simulink model "distributive4"  (R2022b)
settings: Solver=ode8  StartTime=0.0  StopTime=0.25  FixedStep=0.0001  RelTol=1e-3
values from neighbouring files (symbols this model uses):
  A = [a11,0;0,a22]    [distributive3.m]    (also in neurobserver4.m = [1 1;1 2])
  alpha = 0.9e-6    (= 9e-07)    [distributive3.m]
  amp = 80e-6    (= 8e-05)    [distributive3.m]
  angvel = (2*pi)*30    (= 188.495559215)    [distributive3.m]
  B = [b11,0;0,b22]    [distributive3.m]    (also in neurobserver4.m = 1000)
  beta = 0.008    [distributive3.m]
  C = [1,0]    [distributive3.m]
  C_bar = [1,0]    [distributive3.m]    (also in neurobserver4.m = [1,0;0,1])
  d_p = 1.6e-6    (= 1.6e-06)    [distributive3.m]
  fase = 2*pi/10    (= 0.628318530718)    [distributive3.m]
  G = S\C_bar'    [distributive3.m]    (also in neurobserver4.m)
  gamma = 0.008    [distributive3.m]
  Gamma = [0,-B;0 0]    [distributive3.m]    (also in neurobserver4.m = [ 0 , -B ; 0 , 0 ])
  h = legend('Closed-loop response map $(y_d,y)$')    [distributive3.m]    (also in neurobserver4.m = legend('$(y_r,y)$ for $x=7.5$, $f=1Hz$','$(y_r,y)$ for $x=15)
  h_i = 2e-6    (= 2e-06)    [distributive3.m]
  k1 = 7    [distributive3.m]    (also in neurobserver4.m)
  k2 = 7    [distributive3.m]    (also in neurobserver4.m)
  kappa1 = 4e3    (= 4000)    [distributive3.m]    (also in neurobserver4.m = 120)
  L = 20000    [distributive3.m]
  S = [s11,s12;s21,s22]    [distributive3.m]    (also in neurobserver4.m = [1/theta,B/theta^2;B/theta^2,(2*B^2)/theta^3])
  V = learning.V    [neurobserver4.m]
  W = learning.W    [neurobserver4.m]
  x1 = e(2)    [distributive3.m]
  x2 = e(5)    [distributive3.m]
  y_i = -3e-6    (= -3e-06)    [distributive3.m]
undefined symbols (not defined in the file or in its folder): freq, Gamma_c, Y
(part 1 of 3)
settings Model: PacingRate=1000  Creator=mluser  LastModifiedBy=USER
settings OptimizationCC: EnhancedBackFolding=on  PassReuseOutputArgsThreshold=0  MaxStackSize=64  OptimizeBlockOrder=speed  DifferentSizesBufferReuse=on  OptimizationCustomize=off
settings DebuggingCC: SolverPrmCheckMsg=warning  ParameterTunabilityLossMsg=error  ModelReferenceExtraNoncontSigs=warning  UnderSpecifiedDimensionMsg=warning
settings HardwareCC: ProdBitPerPointer=32  ProdBitPerSizeT=32  ProdBitPerPtrDiffT=32  ProdLargestAtomicFloat=None  ProdIntDivRoundTo=Undefined  ProdEndianess=Unspecified  ProdWordSize=32  ProdHWDeviceType=Generic->Unspecified (assume 32-bit Generic)
settings ModelReferenceCC: EnableRefExpFcnMdlSchedulingChecks=on
settings SFSimCC: MATLABDynamicMemAlloc=off
settings RTWCC: Toolchain=Catkin
settings CodeAppCC: ForceParamTrailComments=on  OperatorAnnotations=on
settings GRTTargetCC: TargetLangStandard=C89/C90 (ANSI)

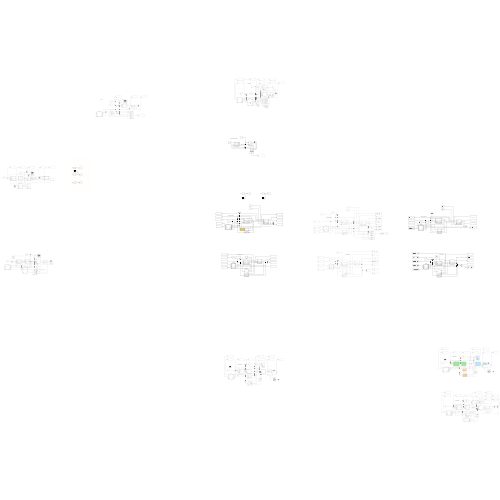
[thumbnail: Simulink's stored preview of the top-level diagram]
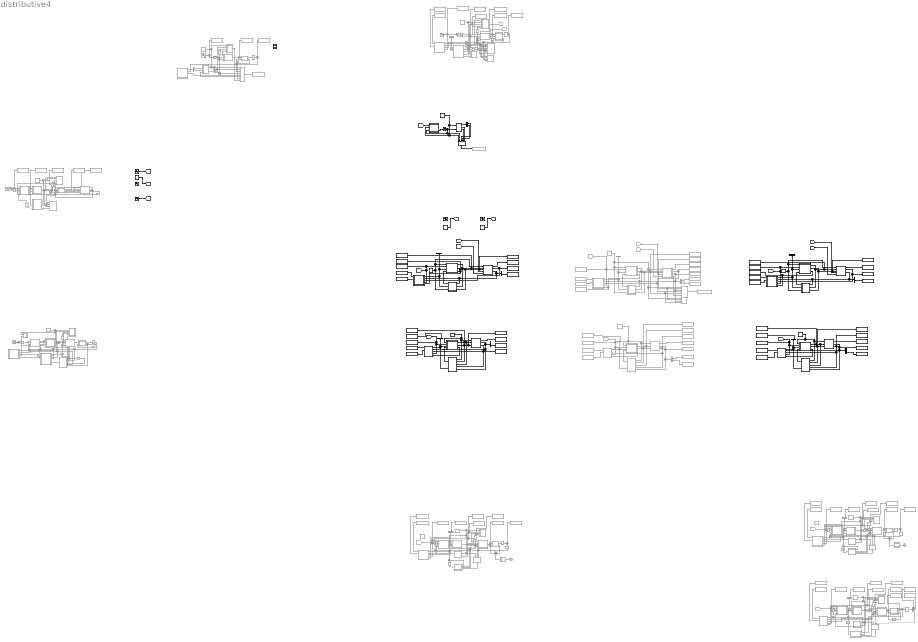
== system distributive4 ==
  note: model
  note: high gain observer
  note: neuroobserver
  note: neuroobserver
  note: inverse model controller
  note: neuroobserver
  note: neuroobserver
  note: no controller
  note: neuroobserver
  note: high gain observer
  note: neuroobserver
  note: high gain observer
  Clock : Clock  Commented=on
  Clock1 : Clock  Commented=on
  Delay3 : Delay  Commented=on  DelayLength=1  InitialCondition=0
  Delay4 : Delay  Commented=on  DelayLength=1  InitialCondition=0
  Demux{1,4,7,10..12,15,21,28} (9 alike) : Demux  Outputs=2
  Demux{2..3,5..6,8..9,23..24,27} (9 alike) : Demux  Commented=on  Outputs=2
  Derivative{2..3,7,12,29..31,35,37} (9 alike) : Derivative  Commented=on
  From1 : From  Commented=on  GotoTag=f10
  From19 : From  Commented=on  GotoTag=A1
  From2 : From  Commented=on  GotoTag=f10
  From21 : From  Commented=on  GotoTag=n
  From22 : From  Commented=on  GotoTag=ny
  From3 : From  Commented=on  GotoTag=ny
  From5 : From  Commented=on  GotoTag=n
  From8 : From  Commented=on  GotoTag=A1
  From9 : From  Commented=on  GotoTag=A1
  IC10 : InitialCondition  Commented=on  Value=0
  IC11 : InitialCondition  Commented=on  Value=h
  IC12 : InitialCondition  Commented=on  Value=Y
  IC13 : InitialCondition  Commented=on  Value=d_p
  IC{6,18..19,33..34} (5 alike) : InitialCondition  Commented=on  Value=h_i
  IC4 : InitialCondition  Commented=on  Value=h
  IC7 : InitialCondition  Commented=on  Value=y_i
  Integrator{2,22,24,35,39} (5 alike) : Integrator  Commented=on  InitialCondition=[0;0]
  Integrator{3,7..9,23,25,36,40} (8 alike) : Integrator  Commented=on
  L1 : Constant  Commented=on  Value=15000
  L5 : Constant  Value=x1
  Mux{1,4,7,23} (4 alike) : Mux  Commented=on  Inputs=8
      settings: DisplayOption=signals
  Mux17 : Mux  Commented=on  Inputs=3
      settings: DisplayOption=signals
  Mux19 : Mux  Commented=on  Inputs=3
      settings: DisplayOption=signals
  Mux2 : Mux  Inputs=6
  Mux22 : Mux  Commented=on  Inputs=3
      settings: DisplayOption=signals
  Mux3 : Mux  Commented=on
      settings: DisplayOption=signals
  Mux30 : Mux  Commented=on
      settings: DisplayOption=signals
  Mux6 : Mux  Commented=on  Inputs=2
  Saturation1 : Saturate  Commented=on  UpperLimit=2000  LowerLimit=-2000
  Saturation4 : Saturate  UpperLimit=20000  LowerLimit=-20000
  Signal Generator : SignalGenerator  WaveForm=sawtooth  Amplitude=amp  Frequency=angvel*10  Units=rad/sec
  Signal Generator1 : SignalGenerator  Amplitude=1*(1e-6)  Frequency=angvel*35  Units=rad/sec
  Signal Generator2 : SignalGenerator  Commented=on  Amplitude=amp  Frequency=angvel  Units=rad/sec
  Signal Generator3 : SignalGenerator  Commented=on  Amplitude=amp  Frequency=angvel  Units=rad/sec
  Signal Generator4 : SignalGenerator  WaveForm=random  Amplitude=1*(1e-6)  Frequency=angvel*20  Units=rad/sec
  Subsystem : Subsystem
  Subsystem1 : Subsystem  Commented=on
  Subsystem10 : Subsystem  Commented=on
  Subsystem11 : Subsystem  Commented=on
  Subsystem12 : Subsystem  Commented=on
      settings: PortSchema="{\"entries\":[{\"content\":{\"sides\":[{\"content\":{\"connectorIds\":[\"Out1\",\"Out2\",\"In1\"]},\"type\":\"ConnectorPlacement.EquallySpacedRectSide\",\"uuid\":\"42746eba-8bba-4a31-9528-796c8edd7bb7\"},{\"content\":{\"connectorIds\":[\"In2\",\"In3\",\"In4\"],\"side\":\"RIGHT\"},\"type\":\"ConnectorPlacement.EquallySpacedRectSide\",\"uuid\":\"7439d13e-5e36-47fa-9d41-de49a9f2c0eb\"},{\"content\":{\"connectorIds\":[],\"side\":\"TOP\"},\"type\":\"ConnectorPlacement.EquallySpacedRectSide\",\"uuid\":\"f708f9c0-884d-4497-944b-57601861f48d\"}]},\"type\":\"ConnectorPlacement.EquallySpacedConnector\",\"uuid\":\"a987a0bb-05be-4e20-b301-42abc30b9f40\"}],\"packageUris\":[\"http://schema.mathworks.com/mf0/Connector/R2020b\"],\"version\":\"1.0\"}"
  Subsystem13 : Subsystem
  Subsystem14 : Subsystem
  Subsystem15 : Subsystem
      settings: PortSchema="{\"entries\":[{\"content\":{\"sides\":[{\"content\":{\"connectorIds\":[\"Out1\",\"Out2\",\"In1\"]},\"type\":\"ConnectorPlacement.EquallySpacedRectSide\",\"uuid\":\"42746eba-8bba-4a31-9528-796c8edd7bb7\"},{\"content\":{\"connectorIds\":[\"In2\",\"In3\",\"In4\"],\"side\":\"RIGHT\"},\"type\":\"ConnectorPlacement.EquallySpacedRectSide\",\"uuid\":\"7439d13e-5e36-47fa-9d41-de49a9f2c0eb\"},{\"content\":{\"connectorIds\":[],\"side\":\"TOP\"},\"type\":\"ConnectorPlacement.EquallySpacedRectSide\",\"uuid\":\"f708f9c0-884d-4497-944b-57601861f48d\"}]},\"type\":\"ConnectorPlacement.EquallySpacedConnector\",\"uuid\":\"a987a0bb-05be-4e20-b301-42abc30b9f40\"}],\"packageUris\":[\"http://schema.mathworks.com/mf0/Connector/R2020b\"],\"version\":\"1.0\"}"
  Subsystem16 : Subsystem
  Subsystem17 : Subsystem
  Subsystem2 : Subsystem
  Subsystem3 : Subsystem
  Subsystem4 : Subsystem
  Subsystem5 : Subsystem
  Subsystem6 : Subsystem
  Subsystem7 : Subsystem
      settings: PortSchema="{\"entries\":[{\"content\":{\"sides\":[{\"content\":{\"connectorIds\":[\"Out1\",\"Out2\",\"In1\"]},\"type\":\"ConnectorPlacement.EquallySpacedRectSide\",\"uuid\":\"42746eba-8bba-4a31-9528-796c8edd7bb7\"},{\"content\":{\"connectorIds\":[\"In2\",\"In3\",\"In4\"],\"side\":\"RIGHT\"},\"type\":\"ConnectorPlacement.EquallySpacedRectSide\",\"uuid\":\"7439d13e-5e36-47fa-9d41-de49a9f2c0eb\"},{\"content\":{\"connectorIds\":[],\"side\":\"TOP\"},\"type\":\"ConnectorPlacement.EquallySpacedRectSide\",\"uuid\":\"f708f9c0-884d-4497-944b-57601861f48d\"}]},\"type\":\"ConnectorPlacement.EquallySpacedConnector\",\"uuid\":\"a987a0bb-05be-4e20-b301-42abc30b9f40\"}],\"packageUris\":[\"http://schema.mathworks.com/mf0/Connector/R2020b\"],\"version\":\"1.0\"}"
  Subsystem8 : Subsystem  Commented=on
  Subsystem9 : Subsystem  Commented=on
  Sum : Sum  Commented=on  Inputs=|++
  Sum1 : Sum  Commented=on  Inputs=|++
  To File1 : ToFile  Commented=on  Filename=train_f10_x1.mat  MatrixName=train
  To File3 : ToFile  Commented=on  Filename=train2_invmod_f1_x3.mat  MatrixName=train
  To File5 : ToFile  Commented=on  Filename=train_mod_20_10.mat  MatrixName=train
  To Workspace : ToWorkspace  Commented=on  VariableName=u_ref  SaveFormat=Timeseries  SampleTime=-1
  To Workspace1 : ToWorkspace  Commented=on  VariableName=y  SaveFormat=Timeseries  SampleTime=-1
  To Workspace10 : ToWorkspace  Commented=on  VariableName=upsilon  SaveFormat=Timeseries  SampleTime=-1
  To Workspace100 : ToWorkspace  Commented=on  VariableName=h_nn3  SaveFormat=Timeseries  SampleTime=-1
  To Workspace101 : ToWorkspace  Commented=on  VariableName=epsilon_y_nn2  SaveFormat=Timeseries  SampleTime=-1
  To Workspace102 : ToWorkspace  Commented=on  VariableName=epsilon_h_nn2  SaveFormat=Timeseries  SampleTime=-1
  To Workspace11 : ToWorkspace  Commented=on  VariableName=h_ref  SaveFormat=Timeseries  SampleTime=-1
  To Workspace12 : ToWorkspace  Commented=on  VariableName=y_ref  SaveFormat=Timeseries  SampleTime=-1
  To Workspace121 : ToWorkspace  VariableName=h_ref_nn3  SaveFormat=Timeseries  SampleTime=-1
  To Workspace122 : ToWorkspace  VariableName=y_ref_nn3  SaveFormat=Timeseries  SampleTime=-1
  To Workspace123 : ToWorkspace  VariableName=u_nn3  SaveFormat=Timeseries  SampleTime=-1
  To Workspace125 : ToWorkspace  VariableName=u_dot_nn3  SaveFormat=Timeseries  SampleTime=-1
  To Workspace126 : ToWorkspace  VariableName=h_nn3  SaveFormat=Timeseries  SampleTime=-1
  To Workspace127 : ToWorkspace  VariableName=epsilon_y_nn3  SaveFormat=Timeseries  SampleTime=-1
  To Workspace129 : ToWorkspace  VariableName=epsilon_h_nn3  SaveFormat=Timeseries  SampleTime=-1
  To Workspace13 : ToWorkspace  Commented=on  VariableName=h_nn  SaveFormat=Timeseries  SampleTime=-1
  To Workspace130 : ToWorkspace  VariableName=y_d_nn3  SaveFormat=Timeseries  SampleTime=-1
  To Workspace131 : ToWorkspace  Commented=on  VariableName=u_nn4  SaveFormat=Timeseries  SampleTime=-1
  To Workspace132 : ToWorkspace  Commented=on  VariableName=y_nn4  SaveFormat=Timeseries  SampleTime=-1
  To Workspace133 : ToWorkspace  Commented=on  VariableName=u_dot_nn4  SaveFormat=Timeseries  SampleTime=-1
  To Workspace135 : ToWorkspace  Commented=on  VariableName=h_nn4  SaveFormat=Timeseries  SampleTime=-1
  To Workspace136 : ToWorkspace  Commented=on  VariableName=epsilon_y_nn4  SaveFormat=Timeseries  SampleTime=-1
  To Workspace137 : ToWorkspace  Commented=on  VariableName=y_L_nn4  SaveFormat=Timeseries  SampleTime=-1
  To Workspace138 : ToWorkspace  Commented=on  VariableName=epsilon_h_nn4  SaveFormat=Timeseries  SampleTime=-1
  To Workspace139 : ToWorkspace  Commented=on  VariableName=y_d_nn4  SaveFormat=Timeseries  SampleTime=-1
  To Workspace14 : ToWorkspace  Commented=on  VariableName=epsilon_y_nn  SaveFormat=Timeseries  SampleTime=-1
  To Workspace140 : ToWorkspace  Commented=on  VariableName=upsilon_nn4  SaveFormat=Timeseries  SampleTime=-1
  To Workspace141 : ToWorkspace  Commented=on  VariableName=h_ref_nn4  SaveFormat=Timeseries  SampleTime=-1
  To Workspace142 : ToWorkspace  Commented=on  VariableName=y_ref_nn4  SaveFormat=Timeseries  SampleTime=-1
  To Workspace147 : ToWorkspace  Commented=on  VariableName=upsilon6  SaveFormat=Timeseries  SampleTime=-1
  To Workspace149 : ToWorkspace  Commented=on  VariableName=y_ref6  SaveFormat=Timeseries  SampleTime=-1
  To Workspace15 : ToWorkspace  Commented=on  VariableName=y_L_nn  SaveFormat=Timeseries  SampleTime=-1
  To Workspace150 : ToWorkspace  Commented=on  VariableName=u6  SaveFormat=Timeseries  SampleTime=-1
  To Workspace151 : ToWorkspace  Commented=on  VariableName=y6  SaveFormat=Timeseries  SampleTime=-1
  To Workspace152 : ToWorkspace  Commented=on  VariableName=u_dot6  SaveFormat=Timeseries  SampleTime=-1
  To Workspace153 : ToWorkspace  Commented=on  VariableName=h6  SaveFormat=Timeseries  SampleTime=-1
  To Workspace154 : ToWorkspace  Commented=on  VariableName=epsilon_y6  SaveFormat=Timeseries  SampleTime=-1
  To Workspace155 : ToWorkspace  Commented=on  VariableName=epsilon_h6  SaveFormat=Timeseries  SampleTime=-1
  To Workspace156 : ToWorkspace  VariableName=y_d_2  SaveFormat=Timeseries  SampleTime=-1
  To Workspace16 : ToWorkspace  Commented=on  VariableName=epsilon_h_nn  SaveFormat=Timeseries  SampleTime=-1
  To Workspace17 : ToWorkspace  Commented=on  VariableName=y_d_nn  SaveFormat=Timeseries  SampleTime=-1
  To Workspace18 : ToWorkspace  Commented=on  VariableName=y_L_nn1  SaveFormat=Timeseries  SampleTime=-1
  To Workspace19 : ToWorkspace  Commented=on  VariableName=y_d_nn1  SaveFormat=Timeseries  SampleTime=-1
  To Workspace2 : ToWorkspace  Commented=on  VariableName=upsilon  SaveFormat=Timeseries  SampleTime=-1
  To Workspace20 : ToWorkspace  Commented=on  VariableName=upsilon_nn  SaveFormat=Timeseries  SampleTime=-1
  To Workspace21 : ToWorkspace  Commented=on  VariableName=upsilon1  SaveFormat=Timeseries  SampleTime=-1
  To Workspace22 : ToWorkspace  Commented=on  VariableName=h_ref1  SaveFormat=Timeseries  SampleTime=-1
  To Workspace23 : ToWorkspace  Commented=on  VariableName=y_ref1  SaveFormat=Timeseries  SampleTime=-1
  To Workspace24 : ToWorkspace  Commented=on  VariableName=u1  SaveFormat=Timeseries  SampleTime=-1
  To Workspace25 : ToWorkspace  Commented=on  VariableName=y1  SaveFormat=Timeseries  SampleTime=-1
  To Workspace26 : ToWorkspace  Commented=on  VariableName=u_dot  SaveFormat=Timeseries  SampleTime=-1
  To Workspace27 : ToWorkspace  Commented=on  VariableName=h  SaveFormat=Timeseries  SampleTime=-1
  To Workspace28 : ToWorkspace  Commented=on  VariableName=epsilon_y  SaveFormat=Timeseries  SampleTime=-1
  To Workspace29 : ToWorkspace  Commented=on  VariableName=epsilon_h  SaveFormat=Timeseries  SampleTime=-1
  To Workspace3 : ToWorkspace  Commented=on  VariableName=h_ref_nn  SaveFormat=Timeseries  SampleTime=-1
  To Workspace30 : ToWorkspace  VariableName=h_nn4  SaveFormat=Timeseries  SampleTime=-1
  To Workspace31 : ToWorkspace  VariableName=epsilon_y_nn4  SaveFormat=Timeseries  SampleTime=-1
  To Workspace33 : ToWorkspace  VariableName=epsilon_h_nn4  SaveFormat=Timeseries  SampleTime=-1
  To Workspace34 : ToWorkspace  VariableName=y_d_nn4  SaveFormat=Timeseries  SampleTime=-1
  To Workspace36 : ToWorkspace  VariableName=y_d_3  SaveFormat=Timeseries  SampleTime=-1
  To Workspace37 : ToWorkspace  VariableName=upsilon_nn4  SaveFormat=Timeseries  SampleTime=-1
  To Workspace38 : ToWorkspace  VariableName=upsilon3  SaveFormat=Timeseries  SampleTime=-1
  To Workspace39 : ToWorkspace  VariableName=h_ref3  SaveFormat=Timeseries  SampleTime=-1
  To Workspace4 : ToWorkspace  Commented=on  VariableName=y_ref_nn  SaveFormat=Timeseries  SampleTime=-1
  To Workspace40 : ToWorkspace  VariableName=y_ref3  SaveFormat=Timeseries  SampleTime=-1
  To Workspace41 : ToWorkspace  VariableName=u3  SaveFormat=Timeseries  SampleTime=-1
  To Workspace43 : ToWorkspace  VariableName=u_dot3  SaveFormat=Timeseries  SampleTime=-1
  To Workspace44 : ToWorkspace  VariableName=h3  SaveFormat=Timeseries  SampleTime=-1
  To Workspace45 : ToWorkspace  VariableName=epsilon_y3  SaveFormat=Timeseries  SampleTime=-1
  To Workspace46 : ToWorkspace  VariableName=epsilon_h3  SaveFormat=Timeseries  SampleTime=-1
  To Workspace47 : ToWorkspace  VariableName=h_ref_nn4  SaveFormat=Timeseries  SampleTime=-1
  To Workspace48 : ToWorkspace  VariableName=upsilon_nn3  SaveFormat=Timeseries  SampleTime=-1
  To Workspace49 : ToWorkspace  VariableName=upsilon2  SaveFormat=Timeseries  SampleTime=-1
  To Workspace5 : ToWorkspace  Commented=on  VariableName=u_nn  SaveFormat=Timeseries  SampleTime=-1
  To Workspace50 : ToWorkspace  VariableName=h_ref2  SaveFormat=Timeseries  SampleTime=-1
  To Workspace51 : ToWorkspace  VariableName=y_ref2  SaveFormat=Timeseries  SampleTime=-1
  To Workspace52 : ToWorkspace  VariableName=u2  SaveFormat=Timeseries  SampleTime=-1
  To Workspace54 : ToWorkspace  VariableName=u_dot2  SaveFormat=Timeseries  SampleTime=-1
  To Workspace55 : ToWorkspace  VariableName=h2  SaveFormat=Timeseries  SampleTime=-1
  To Workspace56 : ToWorkspace  VariableName=epsilon_y2  SaveFormat=Timeseries  SampleTime=-1
  To Workspace57 : ToWorkspace  VariableName=epsilon_h2  SaveFormat=Timeseries  SampleTime=-1
  To Workspace58 : ToWorkspace  VariableName=y_ref_nn4  SaveFormat=Timeseries  SampleTime=-1
  To Workspace59 : ToWorkspace  VariableName=u_nn4  SaveFormat=Timeseries  SampleTime=-1
  To Workspace6 : ToWorkspace  Commented=on  VariableName=y_nn  SaveFormat=Timeseries  SampleTime=-1
  To Workspace60 : ToWorkspace  VariableName=y_nn4  SaveFormat=Timeseries  SampleTime=-1
  To Workspace61 : ToWorkspace  VariableName=u_dot_nn4  SaveFormat=Timeseries  SampleTime=-1
  To Workspace7 : ToWorkspace  Commented=on  VariableName=u_dot_nn  SaveFormat=Timeseries  SampleTime=-1
  To Workspace8 : ToWorkspace  Commented=on  VariableName=u  SaveFormat=Timeseries  SampleTime=-1
  To Workspace85 : ToWorkspace  Commented=on  VariableName=upsilon_nn2  SaveFormat=Timeseries  SampleTime=-1
  To Workspace86 : ToWorkspace  Commented=on  VariableName=h_ref_nn2  SaveFormat=Timeseries  SampleTime=-1
  To Workspace87 : ToWorkspace  Commented=on  VariableName=y_ref_nn2  SaveFormat=Timeseries  SampleTime=-1
  To Workspace88 : ToWorkspace  Commented=on  VariableName=u_nn2  SaveFormat=Timeseries  SampleTime=-1
  To Workspace89 : ToWorkspace  Commented=on  VariableName=y_nn2  SaveFormat=Timeseries  SampleTime=-1
  To Workspace9 : ToWorkspace  Commented=on  VariableName=y  SaveFormat=Timeseries  SampleTime=-1
  To Workspace90 : ToWorkspace  Commented=on  VariableName=u_dot_nn2  SaveFormat=Timeseries  SampleTime=-1
  To Workspace91 : ToWorkspace  Commented=on  VariableName=h_nn2  SaveFormat=Timeseries  SampleTime=-1
  To Workspace92 : ToWorkspace  Commented=on  VariableName=epsilon_y_nn3  SaveFormat=Timeseries  SampleTime=-1
  To Workspace93 : ToWorkspace  Commented=on  VariableName=epsilon_h_nn3  SaveFormat=Timeseries  SampleTime=-1
  To Workspace94 : ToWorkspace  Commented=on  VariableName=upsilon_nn3  SaveFormat=Timeseries  SampleTime=-1
  To Workspace95 : ToWorkspace  Commented=on  VariableName=h_ref_nn3  SaveFormat=Timeseries  SampleTime=-1
  To Workspace96 : ToWorkspace  Commented=on  VariableName=y_ref_nn3  SaveFormat=Timeseries  SampleTime=-1
  To Workspace97 : ToWorkspace  Commented=on  VariableName=u_nn3  SaveFormat=Timeseries  SampleTime=-1
  To Workspace98 : ToWorkspace  Commented=on  VariableName=y_nn3  SaveFormat=Timeseries  SampleTime=-1
  To Workspace99 : ToWorkspace  Commented=on  VariableName=u_dot_nn3  SaveFormat=Timeseries  SampleTime=-1
  dist_vars11 : Subsystem  Commented=on
      settings: PortSchema="{\"entries\":[{\"content\":{\"sides\":[{\"content\":{\"connectorIds\":[\"In1\",\"In2\",\"Out2\",\"Out3\"]},\"type\":\"ConnectorPlacement.EquallySpacedRectSide\",\"uuid\":\"c6804a03-85ed-4e19-a8b2-23b3b91cc999\"},{\"content\":{\"connectorIds\":[\"Out1\"],\"side\":\"RIGHT\"},\"type\":\"ConnectorPlacement.EquallySpacedRectSide\",\"uuid\":\"3893e005-dabd-44b9-aa2f-690b9b6a2b6d\"},{\"content\":{\"connectorIds\":[],\"side\":\"TOP\"},\"type\":\"ConnectorPlacement.EquallySpacedRectSide\",\"uuid\":\"9986ad97-c002-4a16-bb79-a95333cc5799\"}]},\"type\":\"ConnectorPlacement.EquallySpacedConnector\",\"uuid\":\"d796f436-4cc2-4114-998c-ef0d57f68d4d\"}],\"packageUris\":[\"http://schema.mathworks.com/mf0/Connector/R2020b\"],\"version\":\"1.0\"}"
  dist_vars22 : Subsystem  Commented=on
      settings: PortSchema="{\"entries\":[{\"content\":{\"sides\":[{\"content\":{\"connectorIds\":[\"Out1\",\"Out2\",\"Out3\"]},\"type\":\"ConnectorPlacement.EquallySpacedRectSide\",\"uuid\":\"c6804a03-85ed-4e19-a8b2-23b3b91cc999\"},{\"content\":{\"connectorIds\":[\"In1\",\"In2\"],\"side\":\"RIGHT\"},\"type\":\"ConnectorPlacement.EquallySpacedRectSide\",\"uuid\":\"3893e005-dabd-44b9-aa2f-690b9b6a2b6d\"},{\"content\":{\"connectorIds\":[],\"side\":\"TOP\"},\"type\":\"ConnectorPlacement.EquallySpacedRectSide\",\"uuid\":\"9986ad97-c002-4a16-bb79-a95333cc5799\"}]},\"type\":\"ConnectorPlacement.EquallySpacedConnector\",\"uuid\":\"d796f436-4cc2-4114-998c-ef0d57f68d4d\"}],\"packageUris\":[\"http://schema.mathworks.com/mf0/Connector/R2020b\"],\"version\":\"1.0\"}"
  dist_vars23 : Subsystem  Commented=on
      settings: PortSchema="{\"entries\":[{\"content\":{\"sides\":[{\"content\":{\"connectorIds\":[\"Out1\",\"Out2\",\"Out3\"]},\"type\":\"ConnectorPlacement.EquallySpacedRectSide\",\"uuid\":\"c6804a03-85ed-4e19-a8b2-23b3b91cc999\"},{\"content\":{\"connectorIds\":[\"In1\",\"In2\"],\"side\":\"RIGHT\"},\"type\":\"ConnectorPlacement.EquallySpacedRectSide\",\"uuid\":\"3893e005-dabd-44b9-aa2f-690b9b6a2b6d\"},{\"content\":{\"connectorIds\":[],\"side\":\"TOP\"},\"type\":\"ConnectorPlacement.EquallySpacedRectSide\",\"uuid\":\"9986ad97-c002-4a16-bb79-a95333cc5799\"}]},\"type\":\"ConnectorPlacement.EquallySpacedConnector\",\"uuid\":\"d796f436-4cc2-4114-998c-ef0d57f68d4d\"}],\"packageUris\":[\"http://schema.mathworks.com/mf0/Connector/R2020b\"],\"version\":\"1.0\"}"
  dist_vars24 : Subsystem  Commented=on
      settings: PortSchema="{\"entries\":[{\"content\":{\"sides\":[{\"content\":{\"connectorIds\":[\"In1\",\"In2\",\"Out1\",\"Out2\",\"Out3\"]},\"type\":\"ConnectorPlacement.EquallySpacedRectSide\",\"uuid\":\"c6804a03-85ed-4e19-a8b2-23b3b91cc999\"},{\"content\":{\"connectorIds\":[],\"side\":\"RIGHT\"},\"type\":\"ConnectorPlacement.EquallySpacedRectSide\",\"uuid\":\"3893e005-dabd-44b9-aa2f-690b9b6a2b6d\"},{\"content\":{\"connectorIds\":[],\"side\":\"TOP\"},\"type\":\"ConnectorPlacement.EquallySpacedRectSide\",\"uuid\":\"9986ad97-c002-4a16-bb79-a95333cc5799\"}]},\"type\":\"ConnectorPlacement.EquallySpacedConnector\",\"uuid\":\"d796f436-4cc2-4114-998c-ef0d57f68d4d\"}],\"packageUris\":[\"http://schema.mathworks.com/mf0/Connector/R2020b\"],\"version\":\"1.0\"}"
  dist_vars25 : Subsystem  Commented=on
      settings: PortSchema="{\"entries\":[{\"content\":{\"sides\":[{\"content\":{\"connectorIds\":[\"In1\",\"In2\",\"Out1\",\"Out2\",\"Out3\"]},\"type\":\"ConnectorPlacement.EquallySpacedRectSide\",\"uuid\":\"c6804a03-85ed-4e19-a8b2-23b3b91cc999\"},{\"content\":{\"connectorIds\":[],\"side\":\"RIGHT\"},\"type\":\"ConnectorPlacement.EquallySpacedRectSide\",\"uuid\":\"3893e005-dabd-44b9-aa2f-690b9b6a2b6d\"},{\"content\":{\"connectorIds\":[],\"side\":\"TOP\"},\"type\":\"ConnectorPlacement.EquallySpacedRectSide\",\"uuid\":\"9986ad97-c002-4a16-bb79-a95333cc5799\"}]},\"type\":\"ConnectorPlacement.EquallySpacedConnector\",\"uuid\":\"d796f436-4cc2-4114-998c-ef0d57f68d4d\"}],\"packageUris\":[\"http://schema.mathworks.com/mf0/Connector/R2020b\"],\"version\":\"1.0\"}"
  dist_vars3 : Subsystem  Commented=on
      settings: PortSchema="{\"entries\":[{\"content\":{\"sides\":[{\"content\":{\"connectorIds\":[\"In1\",\"In2\",\"Out1\",\"Out2\",\"Out3\"]},\"type\":\"ConnectorPlacement.EquallySpacedRectSide\",\"uuid\":\"c6804a03-85ed-4e19-a8b2-23b3b91cc999\"},{\"content\":{\"connectorIds\":[],\"side\":\"RIGHT\"},\"type\":\"ConnectorPlacement.EquallySpacedRectSide\",\"uuid\":\"3893e005-dabd-44b9-aa2f-690b9b6a2b6d\"},{\"content\":{\"connectorIds\":[],\"side\":\"TOP\"},\"type\":\"ConnectorPlacement.EquallySpacedRectSide\",\"uuid\":\"9986ad97-c002-4a16-bb79-a95333cc5799\"}]},\"type\":\"ConnectorPlacement.EquallySpacedConnector\",\"uuid\":\"d796f436-4cc2-4114-998c-ef0d57f68d4d\"}],\"packageUris\":[\"http://schema.mathworks.com/mf0/Connector/R2020b\"],\"version\":\"1.0\"}"
  dist_vars36 : Subsystem  Commented=on
      settings: PortSchema="{\"entries\":[{\"content\":{\"sides\":[{\"content\":{\"connectorIds\":[\"Out1\",\"Out2\",\"Out3\"]},\"type\":\"ConnectorPlacement.EquallySpacedRectSide\",\"uuid\":\"c6804a03-85ed-4e19-a8b2-23b3b91cc999\"},{\"content\":{\"connectorIds\":[\"In1\",\"In2\"],\"side\":\"RIGHT\"},\"type\":\"ConnectorPlacement.EquallySpacedRectSide\",\"uuid\":\"3893e005-dabd-44b9-aa2f-690b9b6a2b6d\"},{\"content\":{\"connectorIds\":[],\"side\":\"TOP\"},\"type\":\"ConnectorPlacement.EquallySpacedRectSide\",\"uuid\":\"9986ad97-c002-4a16-bb79-a95333cc5799\"}]},\"type\":\"ConnectorPlacement.EquallySpacedConnector\",\"uuid\":\"d796f436-4cc2-4114-998c-ef0d57f68d4d\"}],\"packageUris\":[\"http://schema.mathworks.com/mf0/Connector/R2020b\"],\"version\":\"1.0\"}"
  dist_vars37 : Subsystem  Commented=on
      settings: PortSchema="{\"entries\":[{\"content\":{\"sides\":[{\"content\":{\"connectorIds\":[\"In1\",\"In2\",\"Out2\",\"Out3\",\"Out4\"]},\"type\":\"ConnectorPlacement.EquallySpacedRectSide\",\"uuid\":\"c6804a03-85ed-4e19-a8b2-23b3b91cc999\"},{\"content\":{\"connectorIds\":[\"Out1\"],\"side\":\"RIGHT\"},\"type\":\"ConnectorPlacement.EquallySpacedRectSide\",\"uuid\":\"3893e005-dabd-44b9-aa2f-690b9b6a2b6d\"},{\"content\":{\"connectorIds\":[],\"side\":\"TOP\"},\"type\":\"ConnectorPlacement.EquallySpacedRectSide\",\"uuid\":\"9986ad97-c002-4a16-bb79-a95333cc5799\"}]},\"type\":\"ConnectorPlacement.EquallySpacedConnector\",\"uuid\":\"d796f436-4cc2-4114-998c-ef0d57f68d4d\"}],\"packageUris\":[\"http://schema.mathworks.com/mf0/Connector/R2020b\"],\"version\":\"1.0\"}"
  dist_vars39 : Subsystem  Commented=on
      settings: PortSchema="{\"entries\":[{\"content\":{\"sides\":[{\"content\":{\"connectorIds\":[\"Out1\",\"In1\",\"In2\",\"Out2\",\"Out3\"]},\"type\":\"ConnectorPlacement.EquallySpacedRectSide\",\"uuid\":\"c6804a03-85ed-4e19-a8b2-23b3b91cc999\"},{\"content\":{\"connectorIds\":[\"In3\"],\"side\":\"RIGHT\"},\"type\":\"ConnectorPlacement.EquallySpacedRectSide\",\"uuid\":\"3893e005-dabd-44b9-aa2f-690b9b6a2b6d\"},{\"content\":{\"connectorIds\":[],\"side\":\"TOP\"},\"type\":\"ConnectorPlacement.EquallySpacedRectSide\",\"uuid\":\"9986ad97-c002-4a16-bb79-a95333cc5799\"}]},\"type\":\"ConnectorPlacement.EquallySpacedConnector\",\"uuid\":\"d796f436-4cc2-4114-998c-ef0d57f68d4d\"}],\"packageUris\":[\"http://schema.mathworks.com/mf0/Connector/R2020b\"],\"version\":\"1.0\"}"
  dist_vars4 : Subsystem  Commented=on
      settings: PortSchema="{\"entries\":[{\"content\":{\"sides\":[{\"content\":{\"connectorIds\":[\"In1\",\"Out1\"]},\"type\":\"ConnectorPlacement.EquallySpacedRectSide\",\"uuid\":\"c6804a03-85ed-4e19-a8b2-23b3b91cc999\"},{\"content\":{\"connectorIds\":[],\"side\":\"RIGHT\"},\"type\":\"ConnectorPlacement.EquallySpacedRectSide\",\"uuid\":\"3893e005-dabd-44b9-aa2f-690b9b6a2b6d\"},{\"content\":{\"connectorIds\":[],\"side\":\"TOP\"},\"type\":\"ConnectorPlacement.EquallySpacedRectSide\",\"uuid\":\"9986ad97-c002-4a16-bb79-a95333cc5799\"}]},\"type\":\"ConnectorPlacement.EquallySpacedConnector\",\"uuid\":\"d796f436-4cc2-4114-998c-ef0d57f68d4d\"}],\"packageUris\":[\"http://schema.mathworks.com/mf0/Connector/R2020b\"],\"version\":\"1.0\"}"
  dist_vars40 : Subsystem  Commented=on
      settings: PortSchema="{\"entries\":[{\"content\":{\"sides\":[{\"content\":{\"connectorIds\":[\"In1\",\"In2\",\"Out2\",\"Out3\"]},\"type\":\"ConnectorPlacement.EquallySpacedRectSide\",\"uuid\":\"c6804a03-85ed-4e19-a8b2-23b3b91cc999\"},{\"content\":{\"connectorIds\":[\"Out1\"],\"side\":\"RIGHT\"},\"type\":\"ConnectorPlacement.EquallySpacedRectSide\",\"uuid\":\"3893e005-dabd-44b9-aa2f-690b9b6a2b6d\"},{\"content\":{\"connectorIds\":[],\"side\":\"TOP\"},\"type\":\"ConnectorPlacement.EquallySpacedRectSide\",\"uuid\":\"9986ad97-c002-4a16-bb79-a95333cc5799\"}]},\"type\":\"ConnectorPlacement.EquallySpacedConnector\",\"uuid\":\"d796f436-4cc2-4114-998c-ef0d57f68d4d\"}],\"packageUris\":[\"http://schema.mathworks.com/mf0/Connector/R2020b\"],\"version\":\"1.0\"}"
  dist_vars6 : Subsystem  Commented=on
      settings: PortSchema="{\"entries\":[{\"content\":{\"sides\":[{\"content\":{\"connectorIds\":[\"In1\",\"In2\",\"Out1\",\"Out2\",\"Out3\"]},\"type\":\"ConnectorPlacement.EquallySpacedRectSide\",\"uuid\":\"c6804a03-85ed-4e19-a8b2-23b3b91cc999\"},{\"content\":{\"connectorIds\":[],\"side\":\"RIGHT\"},\"type\":\"ConnectorPlacement.EquallySpacedRectSide\",\"uuid\":\"3893e005-dabd-44b9-aa2f-690b9b6a2b6d\"},{\"content\":{\"connectorIds\":[],\"side\":\"TOP\"},\"type\":\"ConnectorPlacement.EquallySpacedRectSide\",\"uuid\":\"9986ad97-c002-4a16-bb79-a95333cc5799\"}]},\"type\":\"ConnectorPlacement.EquallySpacedConnector\",\"uuid\":\"d796f436-4cc2-4114-998c-ef0d57f68d4d\"}],\"packageUris\":[\"http://schema.mathworks.com/mf0/Connector/R2020b\"],\"version\":\"1.0\"}"
  disturbances : MATLAB Function  Commented=on  TreatAsAtomicUnit=on
  disturbances1 : MATLAB Function  Commented=on  TreatAsAtomicUnit=on
  errors1 : MATLAB Function  Commented=on  TreatAsAtomicUnit=on
  errors11 : MATLAB Function  Commented=on  TreatAsAtomicUnit=on
  errors12 : MATLAB Function  Commented=on  TreatAsAtomicUnit=on
  errors15 : MATLAB Function  TreatAsAtomicUnit=on
  errors16 : MATLAB Function  Commented=on  TreatAsAtomicUnit=on
  errors2 : MATLAB Function  Commented=on  TreatAsAtomicUnit=on
  errors3 : MATLAB Function  Commented=on  TreatAsAtomicUnit=on
  errors4 : MATLAB Function  Commented=on  TreatAsAtomicUnit=on
  errors5 : MATLAB Function  TreatAsAtomicUnit=on
  errors6 : MATLAB Function  Commented=on  TreatAsAtomicUnit=on
  errors7 : MATLAB Function  TreatAsAtomicUnit=on
  errors8 : MATLAB Function  TreatAsAtomicUnit=on
  estimator1 : MATLAB Function  Commented=on  TreatAsAtomicUnit=on
  h_d_ref1 : MATLAB Function  Commented=on  TreatAsAtomicUnit=on
  h_d_ref10 : MATLAB Function  Commented=on  TreatAsAtomicUnit=on
  h_d_ref11 : MATLAB Function  Commented=on  TreatAsAtomicUnit=on
  h_d_ref15 : MATLAB Function  Commented=on  TreatAsAtomicUnit=on
  h_d_ref2 : MATLAB Function  Commented=on  TreatAsAtomicUnit=on
  measurements1 : Subsystem  Commented=on
      settings: PortSchema="{\"entries\":[{\"content\":{\"sides\":[{\"content\":{\"connectorIds\":[]},\"type\":\"ConnectorPlacement.EquallySpacedRectSide\",\"uuid\":\"c6804a03-85ed-4e19-a8b2-23b3b91cc999\"},{\"content\":{\"connectorIds\":[\"Out1\",\"In1\",\"In2\",\"Out2\"],\"side\":\"RIGHT\"},\"type\":\"ConnectorPlacement.EquallySpacedRectSide\",\"uuid\":\"3893e005-dabd-44b9-aa2f-690b9b6a2b6d\"},{\"content\":{\"connectorIds\":[],\"side\":\"TOP\"},\"type\":\"ConnectorPlacement.EquallySpacedRectSide\",\"uuid\":\"9986ad97-c002-4a16-bb79-a95333cc5799\"}]},\"type\":\"ConnectorPlacement.EquallySpacedConnector\",\"uuid\":\"d796f436-4cc2-4114-998c-ef0d57f68d4d\"}],\"packageUris\":[\"http://schema.mathworks.com/mf0/Connector/R2020b\"],\"version\":\"1.0\"}"
  observer : Subsystem
  observer1 : MATLAB Function  Commented=on  TreatAsAtomicUnit=on
  observer10 : MATLAB Function  Commented=on  TreatAsAtomicUnit=on
  observer14 : MATLAB Function  Commented=on  TreatAsAtomicUnit=on
  observer15 : MATLAB Function  Commented=on  TreatAsAtomicUnit=on
  observer2 : Subsystem  Commented=on
  observer3 : Subsystem
  observer9 : MATLAB Function  Commented=on  TreatAsAtomicUnit=on
  system v1 : MATLAB Function  Commented=on  TreatAsAtomicUnit=on
  u3 : Saturate  Commented=on  UpperLimit=500  LowerLimit=-500
  u_ref{1,9..10,14} (4 alike) : Integrator  Commented=on
  u_ref_dot1 : MATLAB Function  Commented=on  TreatAsAtomicUnit=on
  u_ref_dot10 : MATLAB Function  Commented=on  TreatAsAtomicUnit=on
  u_ref_dot11 : MATLAB Function  Commented=on  TreatAsAtomicUnit=on
  u_ref_dot15 : MATLAB Function  Commented=on  TreatAsAtomicUnit=on
  u_ref_dot2 : MATLAB Function  Commented=on  TreatAsAtomicUnit=on
  v1 : MATLAB Function  Commented=on  TreatAsAtomicUnit=on
  v10 : MATLAB Function  Commented=on  TreatAsAtomicUnit=on
  v11 : MATLAB Function  Commented=on  TreatAsAtomicUnit=on
  v15 : MATLAB Function  Commented=on  TreatAsAtomicUnit=on
  v16 : MATLAB Function  Commented=on  TreatAsAtomicUnit=on
  v2 : MATLAB Function  Commented=on  TreatAsAtomicUnit=on
  x1 : Constant  Commented=on  Value=x1
  x10 : Constant  Commented=on  Value=7500
  x{2..3,11,15} (4 alike) : Constant  Commented=on  Value=15000
  x14 : Constant  Value=x1
  x16 : Constant  Commented=on  Value=x1
  x4 : Constant  Commented=on  Value=x2
  x5 : Constant  Value=x2
  x6 : Constant  Value=x1
  x7 : Constant  Value=x2
  y1 : MATLAB Function  Commented=on  TreatAsAtomicUnit=on
  y12 : MATLAB Function  Commented=on  TreatAsAtomicUnit=on
  y13 : MATLAB Function  Commented=on  TreatAsAtomicUnit=on
  y2 : MATLAB Function  Commented=on  TreatAsAtomicUnit=on
  y22 : MATLAB Function  Commented=on  TreatAsAtomicUnit=on
  y23 : MATLAB Function  Commented=on  TreatAsAtomicUnit=on
  y5 : MATLAB Function  Commented=on  TreatAsAtomicUnit=on
  y_1 : InitialCondition  Commented=on  Value=Y
  y_10 : InitialCondition  Commented=on  Value=y_i
  y_2 : InitialCondition  Commented=on  Value=y_i
  y_9 : InitialCondition  Commented=on  Value=y_i
  y_L4 : InitialCondition  Commented=on  Value=[y_i;0]
  y_ref : Sin  Amplitude=amp  Frequency=angvel  Phase=fase  SampleTime=0
  y_ref2 : Sin  Commented=on  Amplitude=amp  Frequency=freq  Phase=fase  SampleTime=0
  y_ref3 : Sin  Commented=on  Amplitude=amp  Frequency=freq  Phase=fase  SampleTime=0
  y_ref4 : Sin  Amplitude=amp  Frequency=angvel*10  Phase=fase  SampleTime=0
  y_ref5 : Sin  Commented=on  Amplitude=80  Frequency=angvel  Phase=fase  SampleTime=0
  y_ref6 : Sin  Amplitude=amp  Frequency=angvel*30  Phase=fase  SampleTime=0
  y_ref7 : Sin  Amplitude=(1e-5)*1  Frequency=angvel*35  Phase=fase  SampleTime=0
  y_ref8 : Sin  Amplitude=1*(1e-5)  Frequency=angvel*20  Phase=0.5  SampleTime=0
  y_ref9 : Sin  Commented=on  Amplitude=amp*4.85e6  Frequency=angvel*10  Phase=fase  SampleTime=0
  Scope : Scope
  wires:
  y2/2(Y_dot) -> Integrator7/1
  Integrator7/1 -> h_d_ref2/4(Y), y2/2(Y)
  y2/1(y) -> IC12/1
  IC10/1 -> dist_vars6/2(u_dot)
  IC11/1 -> v2/3(h_d)
  u_ref_dot2/1(u_ref_dot) -> measurements1/2(u_dot), IC10/1, Integrator8/1
  Derivative3/1 -> h_d_ref2/3(Y_ref_dot)
  measurements1/2(h) -> estimator1/2(h)
  x3/1 -> dist_vars6/1(x), estimator1/1(x)
  measurements1/1(y_L) -> estimator1/4(y_L)
  estimator1/3(h_d_hat) -> u_ref_dot2/2(h_d_hat)
  estimator1/4(d_d_hat) -> IC13/1
  IC13/1 -> h_d_ref2/5(d_d)
  dist_vars6/2(h_d) -> IC11/1
  dist_vars6/1(d_d) -> v2/1(d_d)
  Derivative2/1 -> h_d_ref1/3(Y_ref_dot)
  IC4/1 -> errors2/3(h_d), Mux4/4, v1/3(h_d)
  y_ref2/1 -> errors2/4(y_ref), h_d_ref1/2(Y_ref), Derivative2/1
  u_ref_dot1/1(u_ref_dot) -> Mux4/6, dist_vars3/2(u_dot), u_ref1/1
  y_1/1 -> Mux4/3, errors2/2(y), h_d_ref1/4(Y), observer1/2(y)
  x2/1 -> Derivative7/1, Mux4/1, dist_vars4/1(x), dist_vars3/1(x)
  h_d_ref1/1(h_d_ref) -> u_ref_dot1/1(h_d_ref), errors2/5(h_d_ref)
  y1/1(y) -> y_1/1
  observer1/1(z_hat_dot) -> Integrator2/1
  dist_vars3/1(d_d) -> v1/1(d_d)
  Integrator2/1 -> errors2/1(z_hat), u_ref_dot1/2(z_hat), observer1/1(z_hat)
  y1/2(Y_dot) -> Mux4/7, Integrator3/1
  dist_vars4/1(d_d) -> h_d_ref1/5(d_d)
  u_ref1/1 -> Mux4/2, v1/2(u), h_d_ref1/1(u)
  dist_vars3/2(h_d) -> IC4/1
  v1/1(v) -> y1/1(v)
  Integrator3/1 -> y1/2(Y)
  Mux4/1 -> observer1/3(hZ)
  Derivative7/1 -> Mux4/5
  dist_vars3/3(h_d_dot) -> Mux4/8
  IC6/1 -> system v1/3(h_d), errors4/3(h_d), Mux7/4
  L1/1 -> dist_vars11/1(x), Mux7/1, Derivative12/1, Subsystem1/1(x)
  system v1/1(v) -> To Workspace2/1, y5/1(v)
  y5/1(y) -> IC7/1
  y_ref5/1 -> To Workspace/1, Saturation1/1
  Subsystem1/3(h_d_hat) -> Mux6/2
  dist_vars11/1(h_d_dot) -> Mux7/8
  dist_vars11/2(h_d) -> IC6/1
  dist_vars11/3(d_d) -> system v1/1(d_d)
  Derivative12/1 -> Mux7/5
  Subsystem1/2(y_d_hat) -> Mux6/1
  Saturation1/1 -> Subsystem1/2(u), Mux7/2, system v1/2(u), dist_vars11/2(u)
  Mux7/1 -> To File5/1
  y5/2(Y_dot) -> Mux7/7, Integrator9/1
  Mux6/1 -> errors4/1(z_hat)
  Integrator9/1 -> y5/2(Y)
  Subsystem1/4(u_dot) -> Mux7/6
  IC7/1 -> To Workspace1/1, Mux7/3, errors4/2(y)
  h_d_ref2/1(h_d_ref) -> To Workspace11/1, u_ref_dot2/1(h_d_ref)
  v2/1(v) -> To Workspace10/1, y2/1(v)
  IC12/1 -> To Workspace9/1
  y_ref3/1 -> Derivative3/1, To Workspace12/1, h_d_ref2/2(Y_ref)
  Integrator8/1 -> To Workspace8/1, measurements1/1(u), estimator1/3(u), v2/2(u), h_d_ref2/1(u)
  y_ref/1 -> [f1]
  errors7/2(e_h) -> To Workspace57/1
  errors7/1(e_y) -> To Workspace56/1
  Signal Generator/1 -> [f10]
  y_ref6/1 -> [f30]
  From8/1 -> To Workspace87/1, h_d_ref10/2(Y_ref), Derivative31/1, errors11/4(y_ref)
  errors11/2(e_h) -> To Workspace93/1
  Integrator25/1 -> y12/2(Y)
  IC18/1 -> v10/3(h_d), observer9/3(h_d), errors11/3(h_d)
  dist_vars22/1(d_d) -> h_d_ref10/5(d_d)
  observer9/1(z_hat_dot) -> Integrator24/1
  h_d_ref10/1(h_d_ref) -> errors11/5(h_d_ref), u_ref_dot10/1(h_d_ref)
  x11/1 -> dist_vars24/1(x), u_ref_dot11/3(x), dist_vars23/1(x), Mux17/1
  Derivative29/1 -> h_d_ref11/3(Y_ref_dot)
  u_ref10/1 -> To Workspace97/1, h_d_ref11/1(u), Mux17/2, v11/2(u)
  Integrator23/1 -> y13/2(Y)
  Mux17/1 -> observer10/4(hZ)
  y12/1(y) -> y_9/1
  Integrator22/1 -> errors12/1(z_hat), Demux9/1, u_ref_dot11/2(z_hat), observer10/1(z_hat)
  Delay3/1 -> errors12/2(y), h_d_ref11/4(Y), observer10/2(y), Mux17/3
  y_10/1 -> To Workspace98/1, Delay3/1
  Mux19/1 -> observer9/4(hZ)
  Delay4/1 -> errors11/2(y), h_d_ref10/4(Y), observer9/2(y), Mux19/3
  observer10/1(z_hat_dot) -> Integrator22/1
  Demux8/2 -> To Workspace86/1
  v10/1(v) -> To Workspace85/1, y12/1(v)
  y_9/1 -> To Workspace89/1, Delay4/1
  errors11/1(e_y) -> To Workspace92/1
  dist_vars25/1(d_d) -> v10/1(d_d)
  x10/1 -> dist_vars25/1(x), u_ref_dot10/3(x), dist_vars22/1(x), Mux19/1
  u_ref9/1 -> To Workspace88/1, h_d_ref10/1(u), Mux19/2, v10/2(u)
  Derivative31/1 -> h_d_ref10/3(Y_ref_dot)
  IC19/1 -> v11/3(h_d), observer10/3(h_d), errors12/3(h_d)
  dist_vars23/1(d_d) -> h_d_ref11/5(d_d)
  y13/1(y) -> y_10/1
  h_d_ref11/1(h_d_ref) -> errors12/5(h_d_ref), u_ref_dot11/1(h_d_ref)
  u_ref_dot10/1(u_ref_dot) -> To Workspace90/1, dist_vars25/2(u_dot), u_ref9/1, dist_vars22/2(u_dot)
  u_ref_dot11/1(u_ref_dot) -> To Workspace99/1, dist_vars24/2(u_dot), u_ref10/1, dist_vars23/2(u_dot)
  v11/1(v) -> To Workspace94/1, y13/1(v)
  dist_vars25/2(h_d) -> IC18/1, To Workspace91/1
  Integrator24/1 -> errors11/1(z_hat), Demux8/1, u_ref_dot10/2(z_hat), observer9/1(z_hat)
  errors12/2(e_h) -> To Workspace102/1
  dist_vars24/1(d_d) -> v11/1(d_d)
  From9/1 -> To Workspace96/1, h_d_ref11/2(Y_ref), Derivative29/1, errors12/4(y_ref)
  Demux9/2 -> To Workspace95/1
  dist_vars24/2(h_d) -> IC19/1, To Workspace100/1
  errors12/1(e_y) -> To Workspace101/1
  disturbances/1(delta) -> Sum/2
  Sum/1 -> Integrator25/1
  Clock/1 -> disturbances/1(t)
  y12/2(Y_dot) -> Sum/1
  disturbances1/1(delta) -> Sum1/2
  Clock1/1 -> disturbances1/1(t)
  y13/2(Y_dot) -> Sum1/1
  Sum1/1 -> Integrator23/1
  Mux2/1 -> To File3/1
  Demux15/1 -> Mux2/3
  Demux15/2 -> Mux2/4
  IC33/1 -> observer14/4(h_d), errors6/3(h_d), v15/4(h_d)
  Integrator35/1 -> observer14/1(z_hat), h_d_ref15/4(z_hat), errors6/1(z_hat), Demux24/1, u_ref_dot15/2(z_hat)
  From19/1 -> To Workspace142/1, h_d_ref15/2(y_ref), errors6/4(y_ref), Derivative30/1
  h_d_ref15/1(h_d_ref) -> errors6/5(h_d_ref), u_ref_dot15/1(h_d_ref)
  u_ref_dot15/1(u_ref_dot) -> To Workspace133/1, dist_vars37/2(u_dot), u_ref14/1, dist_vars36/2(u_dot)
  Demux23/2 -> To Workspace139/1
  u_ref14/1 -> To Workspace131/1, h_d_ref15/1(u), v15/3(u), Mux22/2
  dist_vars37/4(h) -> v15/2(h)
  y22/1(y) -> To Workspace132/1, errors6/2(y), observer14/2(y), y_L4/1
  errors6/2(e_h) -> To Workspace138/1
  Demux23/1 -> Mux22/3, To Workspace137/1
  y_L4/1 -> Demux23/1
  x15/1 -> dist_vars37/1(x), u_ref_dot15/3(x), observer14/3(x), dist_vars36/1(x), Mux22/1
  Derivative30/1 -> h_d_ref15/3(y_ref_dot)
  Demux24/2 -> To Workspace141/1
  Integrator36/1 -> y22/2(Y)
  Mux22/1 -> observer14/5(hZ)
  observer14/1(z_hat_dot) -> Integrator35/1
  dist_vars37/2(d_d) -> v15/1(d_d)
  errors6/1(e_y) -> To Workspace136/1
  dist_vars36/3(d_d) -> h_d_ref15/5(d_d)
  v15/1(v) -> To Workspace140/1, y22/1(v)
  Demux21/2 -> To Workspace121/1
  errors15/1(e_y) -> To Workspace127/1
  y22/2(Y_dot) -> Integrator36/1
  [f10] -> Subsystem6/2(y_ref), errors15/4(y_ref), To Workspace122/1
  dist_vars37/3(h_d) -> To Workspace135/1, IC33/1
  errors15/2(e_h) -> To Workspace129/1
  x14/1 -> observer/1(x), Subsystem5/1(x), Subsystem6/1(x)
  errors16/1(e_y) -> To Workspace154/1
  dist_vars39/1(h_d_dot) -> Mux23/8
  v16/1(v) -> To Workspace147/1, y23/1(v)
  Integrator39/1 -> observer15/1(z_hat), Demux27/1, errors16/1(z_hat)
  y23/1(y) -> y_2/1
  dist_vars39/3(h_d) -> IC34/1
  Derivative37/1 -> Mux23/5
  Integrator40/1 -> y23/2(Y)
  observer15/1(z_hat_dot) -> Integrator39/1
  errors16/2(e_h) -> To Workspace155/1
  dist_vars40/2(h_d_dot) -> observer15/4(h_d_dot)
  y_ref9/1 -> errors16/4(y_ref), v16/2(u), Mux30/2, Mux23/2, observer15/3(u), To Workspace150/1, Derivative35/1, To Workspace149/1
  dist_vars40/3(d_d) -> observer15/5(d_d)
  y23/2(Y_dot) -> Mux23/7, Integrator40/1
  dist_vars39/2(d_d) -> v16/1(d_d)
  IC34/1 -> To Workspace153/1, Mux23/4, errors16/3(h_d), v16/3(h_d)
  Derivative35/1 -> dist_vars40/1(u_dot), Mux30/4, Mux23/6, To Workspace152/1, dist_vars39/2(u_dot)
  y_2/1 -> Mux30/3, Mux23/3, errors16/2(y), observer15/2(y), To Workspace151/1
  x16/1 -> Derivative37/1, dist_vars40/2(x), Mux30/1, Mux23/1, dist_vars39/1(x)
  From21/1 -> dist_vars39/3(t)
  Signal Generator4/1 -> [n]
  From22/1 -> y23/3(t)
  Signal Generator1/1 -> [ny]
  Demux28/2 -> To Workspace156/1
  Demux1/2 -> To Workspace130/1
  Saturation4/1 -> Subsystem/2(u), Mux2/2, Subsystem2/3(u)
  L5/1 -> Subsystem/1(x), Mux2/1, Subsystem2/2(x)
  Subsystem/1(Out1) -> Demux15/1
  Subsystem/3(h) -> Mux2/5
  Subsystem/2(Out3) -> Mux2/6
  [f10] -> Subsystem2/1(y_ref)
  Subsystem2/3(u_ref) -> Saturation4/1
  Subsystem3/1(v) -> To Workspace49/1
  [ny] -> Subsystem3/4(ny)
  [n] -> Subsystem3/5(u2)
  Subsystem5/3(h_d) -> observer/4(h_d), To Workspace126/1, errors15/3(h_d)
  Subsystem5/1(v) -> To Workspace48/1
  Subsystem5/2(y) -> observer/5(y), errors15/2(y), Demux1/1
  observer/2(z_hat) -> Subsystem6/3(z_hat), Demux21/1, errors15/1(z_hat)
  Subsystem6/2(u_ref) -> Subsystem5/3(u), To Workspace123/1, observer/2(u)
  Subsystem6/1(u_ref_dot) -> Subsystem5/2(u_dot), observer/3(u_dot), To Workspace125/1
  observer/1(d_d) -> Subsystem6/4(d_d)
  Subsystem6/3(h_d_ref) -> errors15/5(h_d_ref)
  Subsystem3/2(h_d) -> errors7/3(h_d), To Workspace55/1
  [f10] -> To Workspace51/1, Subsystem4/2(Y_ref), errors7/4(y_ref)
  Subsystem3/3(y) -> errors7/2(y), Subsystem7/2(y), Demux28/1
  x6/1 -> Subsystem3/1(x), Subsystem4/1(x), Subsystem7/1(x)
  Subsystem4/2(u_ref) -> Subsystem7/4(u), To Workspace52/1, Subsystem3/3(u)
  Subsystem4/3(h_d_ref) -> errors7/5(h_d_ref), To Workspace50/1
  Subsystem4/1(u_ref_dot) -> To Workspace54/1, Subsystem3/2(u_dot), Subsystem7/3(u_dot)
  Subsystem7/2(z_hat) -> errors7/1(z_hat), Demux4/1, Subsystem4/3(z_hat)
  Subsystem7/1(d_d) -> Subsystem4/4(d_d)
  Subsystem9/1(u_ref_dot) -> To Workspace26/1, Mux1/6, Mux3/4, Subsystem8/2(u_dot), Subsystem12/3(u_dot)
  Subsystem9/2(u_ref) -> Subsystem12/4(u), To Workspace24/1, Mux1/2, Mux3/2, Subsystem8/3(u)
  Subsystem9/3(h_d_ref) -> To Workspace22/1, errors3/5(h_d_ref)
  Mux1/1 -> To File1/1
  observer2/1(d_d) -> Subsystem11/4(d_d)
  Demux2/1 -> To Workspace15/1
  observer2/2(z_hat) -> errors1/1(z_hat), Subsystem11/3(z_hat), Demux3/1
  Subsystem12/1(d_d) -> Subsystem9/4(d_d)
  Subsystem12/2(z_hat) -> errors3/1(z_hat), Demux6/1, Subsystem9/3(z_hat)
  errors3/2(e_h) -> To Workspace29/1
  x1/1 -> Subsystem11/1(x), observer2/1(x), Subsystem10/1(x)
  errors3/1(e_y) -> To Workspace28/1
  Subsystem10/1(v) -> To Workspace20/1
  Subsystem11/2(u_ref) -> observer2/2(u), Subsystem10/3(u), To Workspace5/1
  Subsystem8/4(Y_dot) -> Mux1/7
  Demux2/2 -> To Workspace17/1
  Subsystem8/2(h_d) -> Mux1/4, errors3/3(h_d), To Workspace27/1
  Subsystem10/3(h_d) -> observer2/4(h_d), errors1/3(h_d), To Workspace13/1
  Subsystem11/3(h_d_ref) -> errors1/5(h_d_ref)
  errors1/2(e_h) -> To Workspace16/1
  x4/1 -> Mux3/1, Mux1/1, Subsystem8/1(x), Subsystem9/1(x), Subsystem12/1(x)
  From3/1 -> Subsystem8/4(ny)
  Subsystem11/1(u_ref_dot) -> observer2/3(u_dot), Subsystem10/2(u_dot), To Workspace7/1
  Subsystem8/1(n) -> To Workspace21/1
  Subsystem8/3(y) -> Mux3/3, Mux1/3, errors3/2(y), Subsystem12/2(y), Demux5/1, To Workspace25/1
  Demux5/2 -> To Workspace19/1
  From2/1 -> errors3/4(y_ref), Subsystem9/2(Y_ref), To Workspace23/1
  Demux5/1 -> To Workspace18/1
  Subsystem10/2(y) -> observer2/5(y), Demux2/1, To Workspace6/1
  errors1/1(e_y) -> To Workspace14/1
  From1/1 -> Subsystem11/2(y_ref), errors1/4(y_ref), To Workspace4/1
  Demux3/2 -> To Workspace3/1
  From5/1 -> Subsystem8/5(u2)
  Subsystem17/1(u_ref_dot) -> To Workspace43/1, Subsystem16/2(u_dot), Subsystem15/3(u_dot)
  Subsystem17/2(u_ref) -> Subsystem15/4(u), To Workspace41/1, Subsystem16/3(u)
  Subsystem17/3(h_d_ref) -> errors8/5(h_d_ref), To Workspace39/1
  Subsystem16/2(h_d) -> errors8/3(h_d), To Workspace44/1
  Demux7/2 -> To Workspace34/1
  Subsystem14/2(u_ref) -> observer3/2(u), Subsystem13/3(u), To Workspace59/1
  x5/1 -> Subsystem14/1(x), observer3/1(x), Subsystem13/1(x)
  errors8/1(e_y) -> To Workspace45/1
  Subsystem15/1(d_d) -> Subsystem17/4(d_d)
  observer3/1(d_d) -> Subsystem14/4(d_d)
  errors5/2(e_h) -> To Workspace33/1
  Subsystem14/3(h_d_ref) -> errors5/5(h_d_ref)
  Subsystem13/3(h_d) -> observer3/4(h_d), errors5/3(h_d), To Workspace30/1
  [ny] -> Subsystem16/4(ny)
  x7/1 -> Subsystem16/1(x), Subsystem17/1(x), Subsystem15/1(x)
  observer3/2(z_hat) -> Subsystem14/3(z_hat), Demux10/1, errors5/1(z_hat)
  Demux10/2 -> To Workspace47/1
  errors5/1(e_y) -> To Workspace31/1
  [n] -> Subsystem16/5(u2)
  errors8/2(e_h) -> To Workspace46/1
  [f10] -> Subsystem17/2(Y_ref), To Workspace40/1, errors8/4(y_ref)
  Demux11/2 -> To Workspace36/1
  Subsystem13/1(v) -> To Workspace37/1
  Subsystem15/2(z_hat) -> errors8/1(z_hat), Demux12/1, Subsystem17/3(z_hat)
  Subsystem13/2(y) -> observer3/5(y), Demux7/1, errors5/2(y), To Workspace60/1
  Subsystem16/3(y) -> errors8/2(y), Subsystem15/2(y), Demux11/1
  Subsystem16/1(v) -> To Workspace38/1
  Subsystem14/1(u_ref_dot) -> observer3/3(u_dot), Subsystem13/2(u_dot), To Workspace61/1
  [f10] -> Subsystem14/2(y_ref), errors5/4(y_ref), To Workspace58/1

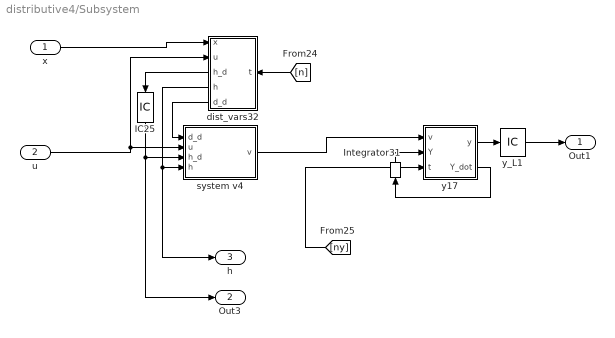
== system distributive4/Subsystem ==
  x : Inport
  u : Inport  Port=2
  IC25 : InitialCondition  Value=h_i
  Integrator31 : Integrator
  dist_vars32 : Subsystem
      settings: PortSchema="{\"entries\":[{\"content\":{\"sides\":[{\"content\":{\"connectorIds\":[\"In1\",\"In2\",\"Out1\",\"Out2\",\"Out3\"]},\"type\":\"ConnectorPlacement.EquallySpacedRectSide\",\"uuid\":\"c6804a03-85ed-4e19-a8b2-23b3b91cc999\"},{\"content\":{\"connectorIds\":[\"In3\"],\"side\":\"RIGHT\"},\"type\":\"ConnectorPlacement.EquallySpacedRectSide\",\"uuid\":\"3893e005-dabd-44b9-aa2f-690b9b6a2b6d\"},{\"content\":{\"connectorIds\":[],\"side\":\"TOP\"},\"type\":\"ConnectorPlacement.EquallySpacedRectSide\",\"uuid\":\"9986ad97-c002-4a16-bb79-a95333cc5799\"}]},\"type\":\"ConnectorPlacement.EquallySpacedConnector\",\"uuid\":\"d796f436-4cc2-4114-998c-ef0d57f68d4d\"}],\"packageUris\":[\"http://schema.mathworks.com/mf0/Connector/R2020b\"],\"version\":\"1.0\"}"
  system v4 : MATLAB Function  TreatAsAtomicUnit=on
  y17 : MATLAB Function  TreatAsAtomicUnit=on
  y_L1 : InitialCondition  Value=[y_i;0]
  Out1 : Outport
  Out3 : Outport  Port=2
  h : Outport  Port=3
  wires:
  IC25/1 -> Out3/1, system v4/3(h_d)
  [n] -> dist_vars32/3(t)
  dist_vars32/1(h_d) -> IC25/1
  dist_vars32/2(h) -> h/1, system v4/4(h)
  y17/1(y) -> y_L1/1
  Integrator31/1 -> y17/2(Y)
  y17/2(Y_dot) -> Integrator31/1
  dist_vars32/3(d_d) -> system v4/1(d_d)
  [ny] -> y17/3(t)
  system v4/1(v) -> y17/1(v)
  u/1 -> dist_vars32/2(u), system v4/2(u)
  y_L1/1 -> Out1/1
  x/1 -> dist_vars32/1(x)

== system distributive4/Subsystem1 ==
  x : Inport
  u : Inport  Port=2
  Derivative1 : Derivative
  Integrator2 : Integrator
  estimator : MATLAB Function  TreatAsAtomicUnit=on
  measurements : Subsystem
      settings: PortSchema="{\"entries\":[{\"content\":{\"sides\":[{\"content\":{\"connectorIds\":[]},\"type\":\"ConnectorPlacement.EquallySpacedRectSide\",\"uuid\":\"c6804a03-85ed-4e19-a8b2-23b3b91cc999\"},{\"content\":{\"connectorIds\":[\"Out1\",\"In1\",\"Out2\"],\"side\":\"RIGHT\"},\"type\":\"ConnectorPlacement.EquallySpacedRectSide\",\"uuid\":\"3893e005-dabd-44b9-aa2f-690b9b6a2b6d\"},{\"content\":{\"connectorIds\":[],\"side\":\"TOP\"},\"type\":\"ConnectorPlacement.EquallySpacedRectSide\",\"uuid\":\"9986ad97-c002-4a16-bb79-a95333cc5799\"}]},\"type\":\"ConnectorPlacement.EquallySpacedConnector\",\"uuid\":\"d796f436-4cc2-4114-998c-ef0d57f68d4d\"}],\"packageUris\":[\"http://schema.mathworks.com/mf0/Connector/R2020b\"],\"version\":\"1.0\"}"
  d_d_hat : Outport
  y_d_hat : Outport  Port=2
  h_d_hat : Outport  Port=3
  u_dot : Outport  Port=4
  wires:
  estimator/1(y_d_hat) -> y_d_hat/1
  estimator/4(d_d_hat) -> d_d_hat/1
  u/1 -> estimator/2(u), Derivative1/1
  Integrator2/1 -> estimator/1(h)
  Derivative1/1 -> u_dot/1, estimator/3(u_dot)
  x/1 -> estimator/4(x)
  estimator/2(h_dot) -> Integrator2/1
  estimator/3(h_d_hat) -> h_d_hat/1
